simulink model "SimpleScenarioAndSensorModel3DSimulation"  (R2020a)
settings: Solver=FixedStepAuto  StartTime=0.0  StopTime=60.0  FixedStep=Auto  RelTol=1e-3
undefined symbols (not defined in the file or in its folder): f
libraries: etargetslib x3, sim3dautolib x3, instrumentlib x3, simulink_extras x2, vehdynlibsteering x1, mpcadaslib x1, sim3dlib x1, autolibshared x1
settings Model: EnablePacing=on  Creator=The MathWorks, Inc.  LastModifiedBy=javot
settings DebuggingCC: SymbolicDimsDataTypeCodeGenerationDiagnostic=none

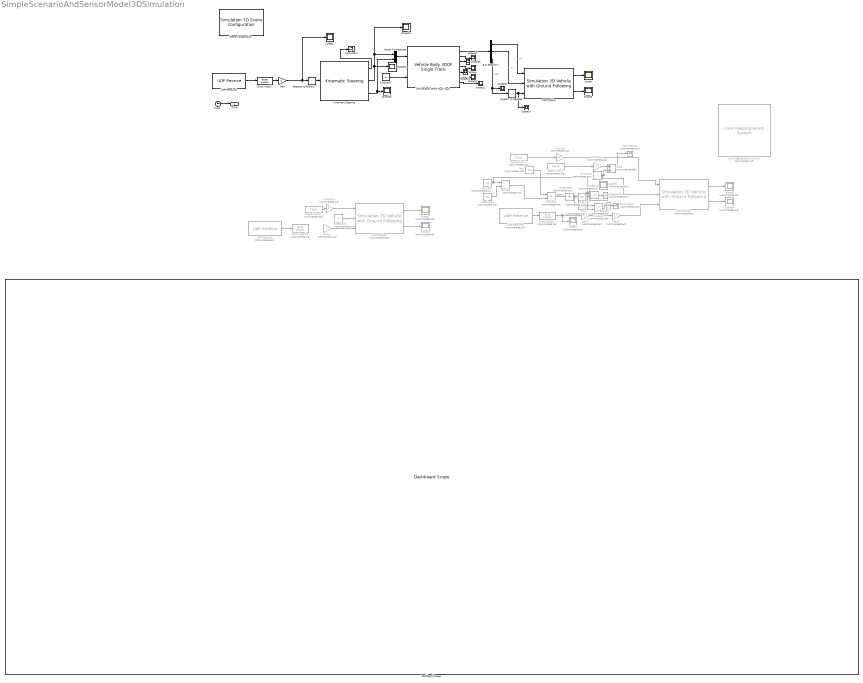
== system SimpleScenarioAndSensorModel3DSimulation ==
  Add1 : Sum  Commented=on
  Bus Selector1 : BusSelector  OutputSignals=InertFrm.Geom.Disp.X,InertFrm.Geom.Disp.Y,InertFrm.Cg.Ang.psi
  Byte Unpack : etargetslib/Byte Unpack  dimensions={[1]}  datatypes={'double'}  byteAlign=1
  Byte Unpack1 : etargetslib/Byte Unpack  Commented=on  dimensions={[1]}  datatypes={'double'}  byteAlign=1
  Byte Unpack2 : etargetslib/Byte Unpack  Commented=on  dimensions={[1]}  datatypes={'double'}  byteAlign=1
  CAPTMobile : sim3dautolib/Simulation 3D Vehicle with Ground Following  Priority=-1  PassVehMesh=Sport utility vehicle  VehColor=Blue  InitialPos=[10, 0, 0]  InitialRot=[0, 0, 90]  ActorName=CAPTMobile  SampleTime=-1  ActorType=SimulinkVehicle  ID=C  aMode=3  ActorTag=CAPTMobile  CoordinateScheme=ISO  TransformOutportEnabled=on
      settings: SourceProductBaseCode=DR,VE
  CAPTMobile1 : sim3dautolib/Simulation 3D Vehicle with Ground Following  Priority=-1  Commented=on  PassVehMesh=Sport utility vehicle  VehColor=Blue  InitialPos=[10, 0, 0]  InitialRot=[0, 0, 90]  ActorName=SimulinkVehicle1  SampleTime=-1  ActorType=SimulinkVehicle  ID=1  aMode=3  ActorTag=SimulinkVehicle1  CoordinateScheme=ISO  TransformOutportEnabled=on
      settings: SourceProductBaseCode=DR,VE
  CAPTMobile2 : sim3dautolib/Simulation 3D Vehicle with Ground Following  Priority=-1  Commented=on  PassVehMesh=Sport utility vehicle  VehColor=Blue  InitialPos=[0, 0, 0]  InitialRot=[0, 0, 90]  ActorName=SimulinkVehicle2  SampleTime=-1  ActorType=SimulinkVehicle  ID=2  aMode=3  ActorTag=SimulinkVehicle2  CoordinateScheme=ISO  TransformOutportEnabled=on
      settings: SourceProductBaseCode=DR,VE
  Clock : Clock
  Constant3 : Constant  Commented=on  Value=0
  Constant4 : Constant  Commented=on  Value=0
  Constant7 : Constant  Value=5
  Cos1 : Trigonometry  Commented=on  Operator=cos
  Dashboard Scope : DashboardScope
  Degrees to Radians : simulink_extras/Transformations/Degrees to Radians
  Digital Clock1 : DigitalClock  Commented=on  SampleTime=0.01
  Digital Clock2 : DigitalClock  Commented=on  SampleTime=0.01
  Digital Clock3 : DigitalClock  Commented=on  SampleTime=0.01
  Divide1 : Product  Commented=on  Inputs=*/
  Gain : Gain  Gain=-1
  Gain2 : Gain  Commented=on  Gain=-1
  Gain3 : Gain  Commented=on
  Gain4 : Gain  Commented=on  Gain=-1
  Integrator3 : Integrator  Commented=on
  Integrator4 : Integrator  Commented=on
  Integrator5 : Integrator  Commented=on
  Kinematic Steering : vehdynlibsteering/Kinematic Steering  StrgType=Rack and pinion  StrgRatioType=Constant  Loc=Front  NrmlFctr=0.01  TrckWdth=1  WhlBase=1.524  Db=0  StrgRng=1.25*pi  StrgAngBpts="[-6.2832   -5.0265   -3.7699   -2.5133   -1.2566         0    1.2566    2.5133    3.7699    5.0265    6.2832]"  StrgRatioTbl=|  StrgRatio=10  StrgArmLngth=0.1  RckCsLngth=0.5  TieRodLngth=0.248  D=0.2  PnnRadius=0.0057  PnnRadiusTbl="[0.0055    0.0055    0.0056    0.0057    0.0058    0.0057    0.0057    0.0057    0.0056    0.0055    0.0055]"  RodLngth=0.1  ParaArmLngth=0.9  aMode=2
      | [13.5000   13.3750   13.2500   13.1250   13.0000   13.0000   13.0000   13.1250   13.2500   13.3750   13.5000
      | ]
  Lane Keeping Assist System : mpcadaslib/Lane Keeping Assist System  Commented=on  ModelType=Use vehicle parameters  VehicleMass=1575  VehicleYawInertia=2875  LengthToFront=1.2  LengthToRear=1.6  FrontTireStiffness=19000  RearTireStiffness=33000  EgoModelMatrixA=[-4.4021 ,-12.4603;1.3913,-5.1868]  EgoModelMatrixB=[24.1270;15.8609]  EgoModelMatrixC=[1,0;0,1]  InitialLongVel=15  TransportLag=0  MinSteering=-0.26  umin_ext=off  MaxSteering=0.26  umax_ext=off  Ts=0.1  PredictionHorizon=10  ControllerBehavior=0.5  suboptimal=off  maxiter=10  datatypeopt=double  optmode=off  trackmode=off
      settings: SourceProductBaseCode=MP
  Multiply1 : Gain  Commented=on  Gain=5
  Multiply2 : Gain  Commented=on  Gain=10
  Multiply3 : Gain  Commented=on  Gain=0
  Product3 : Product  Commented=on
  Product4 : Product  Commented=on
  Product5 : Product  Commented=on
  Radians to Degrees : simulink_extras/Transformations/Radians to Degrees
  Scene Configuration : sim3dlib/Simulation 3D Scene Configuration  Priority=0  ProjectFormat=Default Scenes  SceneDesc=Straight road  ProjectName=VehicleSimulation.exe  ScenePath=/Game/Maps/HwStrght  vehTagList={'CAPTMobile';'Scene Origin';'SimulinkVehicle1';'SimulinkVehicle2'}  vehTag=CAPTMobile  OpVisEn=off  Ts=1/100  EnableWindow=on  sensorTag=MainCamera2  sensorId=2  sensorName=MainCamera2  mountLoc=Origin  offsetFlag=off  tmountOffset=[0, 0, 0]  rmountOffset=[0, 0, 0]  HorizontalResolution=1280  VerticalResolution=720  HorizontalFOV=60  mountPoint=[0 0 0]  mountOrientation=[0 0 0]  aMode=3  ID=2
      settings: SourceProductBaseCode=DR,VE
  Scope{,1,4..5,10..19} (14 alike) : Scope
  Scope{2..3,6..9} (6 alike) : Scope  Commented=on
  Sin1 : Trigonometry  Commented=on
  Tan1 : Trigonometry  Commented=on  Operator=tan
  Terminator : Terminator
  Terminator3 : Terminator  Commented=on
  Terminator4 : Terminator  Commented=on
  UDP Receive1 : instrumentlib/UDP Receive  Commented=on  Host=localhost  Port=55001  LocalPort=55001  EnablePortSharing=off  GetLatestData=on  DataSize=8  DataType=uint8  ASCIIFormatting=%f,  Terminator=LF  ByteOrder=BigEndian  EnableBlockingMode=on  Timeout=10  SampleTime=0.01  LocalAddress=134.105.60.99
  UDP Receive2 : instrumentlib/UDP Receive  Host=localhost  Port=5006  LocalPort=5006  EnablePortSharing=off  GetLatestData=on  DataSize=8  DataType=uint8  ASCIIFormatting=%f,  Terminator=LF  ByteOrder=LittleEndian  EnableBlockingMode=on  Timeout=10  SampleTime=0.01  LocalAddress=127.0.0.1
  UDP Receive3 : instrumentlib/UDP Receive  Commented=on  Host=localhost  Port=55001  LocalPort=55001  EnablePortSharing=off  GetLatestData=on  DataSize=8  DataType=uint8  ASCIIFormatting=%f,  Terminator=LF  ByteOrder=BigEndian  EnableBlockingMode=on  Timeout=10  SampleTime=0.01  LocalAddress=134.105.60.99
  Vector Concatenate : Concatenate
  Vehicle Body 3DOF Dual Track : autolibshared/Vehicle Body 3DOF Single Track  trackMode=Dual  inputMode=External longitudinal velocity  frontSteerMode=on  rearSteerMode=off  windMode=off  muMode=off  extFMode=off  extMMode=off  extXo=off  extpsio=off  extxdoto=off  extro=off  extYo=off  extTamb=off  extydoto=off  aMode=2  NF=2  NR=2  m=2000  a=1.4  b=1.6  h=0.35  X_o=0  xdot_o=0  CalphaMode=off  sigmaMode=on  d=0  w=[1.4,1.4]  Cy_f=12e3  Cy_r=11e3  sigma_f=.1  sigma_r=.1  alpha_f_brk=[-.1 .1]  Cy_f_data=[-9e3 9e3]  alpha_r_brk=[-.1 .1]  Cy_r_data=[-9e3 9e3]  Y_o=0  ydot_o=0  Izz=4000  psi_o=0  r_o=0  Af=2  Cd=.3  Cl=.1  Cpm=.1  beta_w=[0:0.01:0.3]  Cs=[0:0.03:0.9]  Cym=[0:0.01:0.3]  Pabs=101325  Tair=273  g=9.81  mu=1  xdot_tol=.01  Fznom=5000  Fxtire_sat=7e4  Fytire_sat=7e4  longOff=0  latOff=0  vertOff=0  wrapAng=off
      settings: SourceProductBaseCode=PW,MT,VE,VP
  car_vel1 : Constant  Commented=on  Value=10
  wheelbase1 : Constant  Commented=on  Value=0.1
  time : Outport
  wires:
  CAPTMobile/1 -> Scope/1
  CAPTMobile/2 -> Scope5/1
  Clock/1 -> time/1
  Add1/1 -> Terminator4/1
  Product5/1 -> Integrator5/1
  Gain3/1 -> CAPTMobile1/3
  wheelbase1/1 -> Divide1/2
  Integrator5/1 -> Terminator3/1
  Product3/1 -> Integrator3/1  "psi_dot"
  Integrator3/1 -> Sin1/1, Cos1/1
  Sin1/1 -> Product5/1
  Digital Clock3/1 -> Multiply3/1
  Digital Clock2/1 -> Multiply2/1
  Product4/1 -> Integrator4/1
  Multiply2/1 -> CAPTMobile1/1
  Constant3/1 -> Add1/2, CAPTMobile1/2
  Cos1/1 -> Product4/2
  Multiply3/1 -> Add1/1
  Tan1/1 -> Product3/1
  CAPTMobile1/1 -> Scope6/1
  UDP Receive3/1 -> Byte Unpack1/1
  car_vel1/1 -> Product5/2, Product4/1, Divide1/1
  CAPTMobile1/2 -> Scope9/1
  Integrator4/1 -> Scope8/1
  Divide1/1 -> Product3/2
  Gain2/1 -> Gain3/1
  Byte Unpack1/1 -> Scope7/1, Gain2/1
  CAPTMobile2/2 -> Scope2/1
  CAPTMobile2/1 -> Scope3/1
  Gain4/1 -> CAPTMobile2/3
  Constant4/1 -> CAPTMobile2/2
  Multiply1/1 -> CAPTMobile2/1
  Digital Clock1/1 -> Multiply1/1
  UDP Receive1/1 -> Byte Unpack2/1
  UDP Receive2/1 -> Byte Unpack/1
  Byte Unpack/1 -> Gain/1
  Vehicle Body 3DOF Dual Track/2 -> Scope17/1
  Bus Selector1/2 -> CAPTMobile/2  "<Y>"
  Vehicle Body 3DOF Dual Track/3 -> Scope16/1
  Vehicle Body 3DOF Dual Track/5 -> Scope13/1
  Vehicle Body 3DOF Dual Track/6 -> Scope11/1
  Vehicle Body 3DOF Dual Track/7 -> Scope12/1
  Constant7/1 -> Vehicle Body 3DOF Dual Track/2
  Vehicle Body 3DOF Dual Track/1 -> Bus Selector1/1
  Vehicle Body 3DOF Dual Track/4 -> Scope4/1
  Bus Selector1/1 -> CAPTMobile/1  "<X>"
  Bus Selector1/3 -> Radians to Degrees/1, Scope18/1  "<psi>"
  Kinematic Steering/1 -> Terminator/1
  Degrees to Radians/1 -> Kinematic Steering/1
  Gain/1 -> Scope1/1, Degrees to Radians/1
  Radians to Degrees/1 -> Scope14/1, CAPTMobile/3
  Kinematic Steering/3 -> Vector Concatenate/2, Scope15/1
  Vector Concatenate/1 -> Vehicle Body 3DOF Dual Track/1
  Kinematic Steering/2 -> Vector Concatenate/1, Scope10/1, Scope19/1
